simulink model "Inverse_Dynamics_Control_SCARA_trial1"  (R2019b)
settings: Solver=VariableStepAuto  StartTime=0.0  StopTime=20  RelTol=1e-3
undefined symbols (not defined in the file): DiscIntNeverNeededParam, q0, q0_dot, Tc
settings Model: Creator=manth  LastModifiedBy=manth

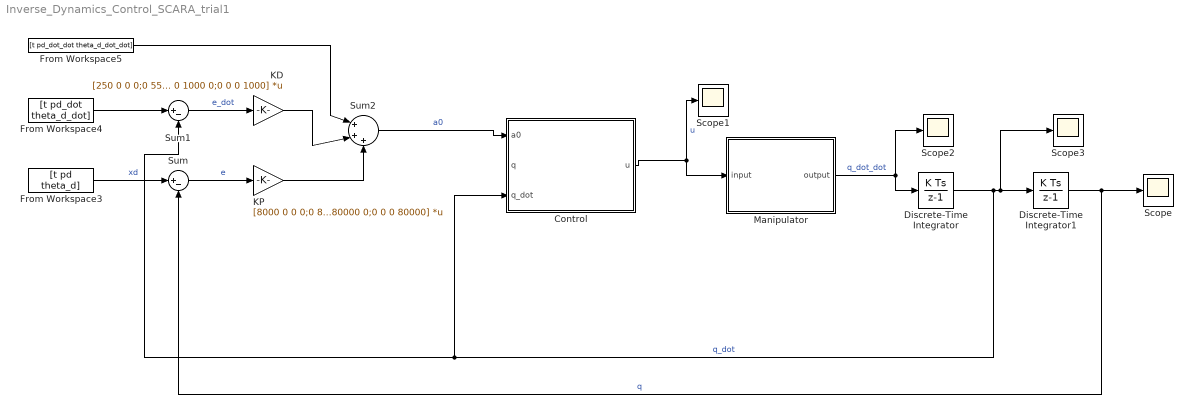
== system Inverse_Dynamics_Control_SCARA_trial1 ==
  Control : MATLAB Function  TreatAsAtomicUnit=on
  Discrete-Time Integrator : DiscreteIntegrator  InitialCondition=q0_dot  SampleTime=Tc  ICPrevOutput=DiscIntNeverNeededParam  ICPrevScaledInput=DiscIntNeverNeededParam
  Discrete-Time Integrator1 : DiscreteIntegrator  InitialCondition=q0  SampleTime=Tc  ICPrevOutput=DiscIntNeverNeededParam  ICPrevScaledInput=DiscIntNeverNeededParam
  From Workspace3 : FromWorkspace  VariableName=[t pd theta_d]  SampleTime=Tc
  From Workspace4 : FromWorkspace  VariableName=[t pd_dot theta_d_dot]  SampleTime=Tc
  From Workspace5 : FromWorkspace  VariableName=[t pd_dot_dot theta_d_dot_dot]  SampleTime=Tc
  KD : Gain  Gain=[250 0 0 0;0 550 0 0;0 0 1000 0;0 0 0 1000]  Multiplication=Matrix(K*u) (u vector)
  KP : Gain  Gain=[8000 0 0 0;0 8000 0 0;0 0 80000 0;0 0 0 80000]  Multiplication=Matrix(K*u) (u vector)
  Manipulator : MATLAB Function  TreatAsAtomicUnit=on
  Scope{,1..3} (4 alike) : Scope
  Sum : Sum  Inputs=|+-
  Sum1 : Sum  Inputs=|+-
  Sum2 : Sum  Inputs=|+++
  wires:
  Manipulator/1(output) -> Discrete-Time Integrator/1, Scope2/1  "q_dot_dot"
  Discrete-Time Integrator/1 -> Discrete-Time Integrator1/1, Scope3/1, Sum1/2, Control/3(q_dot)  "q_dot"
  Discrete-Time Integrator1/1 -> Sum/2, Scope/1  "q"
  Sum2/1 -> Control/1(a0)  "a0"
  Control/1(u) -> Manipulator/1(input), Scope1/1  "u"
  From Workspace4/1 -> Sum1/1
  Sum/1 -> KP/1  "e"
  From Workspace5/1 -> Sum2/1
  KP/1 -> Sum2/3
  From Workspace3/1 -> Sum/1  "xd"
  Sum1/1 -> KD/1  "e_dot"
  KD/1 -> Sum2/2

== matlab function Inverse_Dynamics_Control_SCARA_trial1/Control ==
  data: a0 input; q input; u output; q_dot input
function u  = Control(a0,q,q_dot)
   theta2=q(2,:);
    theta1_dot=q(5,:);
    theta2_dot=q(6,:);
    d3_dot=q(7,:);
    theta4_dot=q(8,:);
    m_l2 = 25;
    m_l3 = 10;
    m_l4 = 0;
    l_2 = 0.25;
    k_r1 = 1;
    k_r2 = 1;
    k_r3 = 50;
    k_r4 = 20;
    g = 9.8;
    Fv_1 = 0.0001;
    Fv_2 = 0.0001;
    Fv_3 = 0.01;
    Fv_4 = 0.005;
    C_cap=[(-l_2*m_l2*sin(theta2)-0.5*(m_l4+m_l3)*sin(theta2))/2*theta2_dot (-l_2*m_l2*sin(theta2)-0.5*(m_l4+m_l3)*sin(theta2))/2*(theta1_dot+theta2_dot) 0 0;
    -(-l_2*m_l2*sin(theta2)-0.5*(m_l4+m_l3)*sin(theta2))/2*theta1_dot 0 0 0; 0 0 0 0; 0 0 0 0];
    G = [0; 0; -(m_l3+m_l4)*g; 0];
    
    
        theta2=input(2,:);
    y1=input(5,:);
    y2=input(6,:);
    y3=input(7,:);    
    y4=input(8,:);
    m_l1 = 25;
    m_l2 = 25;
    m_l3 = 10;
    m_l4 = 0;
    I_l1 = 5; 
    I_l2 = 5;
    I_l4 = 1;
    I_m1 = 0.0001;
    I_m2 = 0.0001; 
    I_m3 = 0.01;
    I_m4 = 0.005;
    l_1 = 0.25;
    l_2 = 0.25;
    k_r1 = 1;
    k_r2 = 1;
    k_r3 = 50;
    k_r4 = 20;
    g = 9.8;
    b11=l_1^2*m_l1+(0.25+l_2^2+l_2*cos(theta2))*m_l2+(0.5+0.5*cos(theta2))*(m_l3+m_l4)+I_l1+I_l2+I_l4+I_m1*k_r1^2+I_m2+I_m3+I_m4;
    b12=(0.5*l_2*cos(theta2)+l_2^2)*m_l2+(0.25+0.25*cos(theta2))*(m_l3+m_l4)+I_l2+I_l4+I_m2*k_r2++I_m3+I_m4;
    b13=-k_r3*I_m3;
    b14=k_r4*I_m4+I_l4;
    b21=b12;
    b22=l_2^2*m_l2+0.25*(m_l4+m_l3)+I_l2+I_l4+I_m2*k_r2^2+I_m4+I_m3;
    b23=-k_r3*I_m3;
    b24=k_r4*I_m4+I_l4;
    b31=b13;
    b32=b23;
    b33=I_m3*k_r3^2+m_l3+m_l4;
    b34=0;
    b41=b14;
    b42=b24;
    b43=b34;
    b44=I_m4*k_r4^2+I_l4;
    B_cap=[b11 b12 b13 b14; b21 b22 b23 b24; b31 b32 b33 b34; b41 b42 b43 b44];
    
    
u=B_cap*a0+G+C_cap*q_dot;
  
end

== matlab function Inverse_Dynamics_Control_SCARA_trial1/Manipulator ==
  data: input input; output output
function output = Manipulator(input)
% Part 2 manipulator
    theta1 = input(1,:);
    theta2 = input(2,:);
    d3 = input(3,:);
    theta4 = input(4,:);
    theta1_dot = input(5,:);
    theta2_dot = input(6,:);
    d3_dot = input(7,:);
    theta4_dot = input(8,:);
    u1 = input(9,:);
    u2 = input(10,:);
    u3 = input(11,:);
    u4 = input(12,:);
    m_l1 = 25;
    m_l2 = 25;
    m_l3 = 10;
    m_l4 = 5;
    I_l1 = 5;
    I_l2 = 5;
    I_l4 = 1;
    I_m1 = 0.0001;
    I_m2 = 0.0001;
    I_m3 = 0.01;
    I_m4 = 0.005;
    l_1 = 0.25;
    l_2 = 0.25;
    k_r1 = 1;
    k_r2 = 1;
    k_r3 = 50;
    k_r4 = 20;
    g = 9.8;
    Fv_1 = 0.0001;
    Fv_2 = 0.0001;
    Fv_3 = 0.01;
    Fv_4 = 0.005;
    
    b11=l_1^2*m_l1+(0.25+l_2^2+l_2*cos(theta2))*m_l2+(0.5+0.5*cos(theta2))*(m_l3+m_l4)+I_l1+I_l2+I_l4+I_m1*k_r1^2+I_m2+I_m3+I_m4;
    b12=(0.5*l_2*cos(theta2)+l_2^2)*m_l2+(0.25+0.25*cos(theta2))*(m_l3+m_l4)+I_l2+I_l4+I_m2*k_r2++I_m3+I_m4;
    b13=-k_r3*I_m3;
    b14=k_r4*I_m4+I_l4;
    b21=b12;
    b22=l_2^2*m_l2+0.25*(m_l4+m_l3)+I_l2+I_l4+I_m2*k_r2^2+I_m4+I_m3;
    b23=-k_r3*I_m3;
    b24=k_r4*I_m4+I_l4;
    b31=b13;
    b32=b23;
    b33=I_m3*k_r3^2+m_l3+m_l4;
    b34=0;
    b41=b14;
    b42=b24;
    b43=b34;
    b44=I_m4*k_r4^2+I_l4;
    B=[b11 b12 b13 b14; b21 b22 b23 b24; b31 b32 b33 b34; b41 b42 b43 b44];
    C=[(-l_2*m_l2*sin(theta2)-0.5*(m_l4+m_l3)*sin(theta2))/2*theta2_dot (-l_2*m_l2*sin(theta2)-0.5*(m_l4+m_l3)*sin(theta2))/2*(theta1_dot+theta2_dot) 0 0;
    -(-l_2*m_l2*sin(theta2)-0.5*(m_l4+m_l3)*sin(theta2))/2*theta1_dot 0 0 0; 0 0 0 0; 0 0 0 0];
    G = [0; 0; -(m_l3+m_l4)*g; 0];
    F = diag([k_r1^2*Fv_1 k_r2^2*Fv_2 k_r3^2*Fv_3 k_r4^2*Fv_4]);
    
    tou = [u1 u2 u3 u4]';
    tou_1 = C*[theta1_dot theta2_dot d3_dot theta4_dot]'+F*[theta1_dot theta2_dot d3_dot theta4_dot]'+G;
    
    q_dot_dot = inv(B)*(tou-tou_1);
    
    output = q_dot_dot;
    % output(2) = q_dot_dot(2);
    % output(3) = q_dot_dot(3);
    % output(4) = q_dot_dot(4);
end
